simulink model "DiscreteDiscrete"  (R2017b)
settings: Solver=VariableStepAuto  StartTime=0.0  StopTime=10.0  RelTol=1e-3
values from neighbouring files (symbols this model uses):
  kd = double(kd)    [DiscreteDiscreteMatlab.m]    (also in P_I_D.m = eval(S.kd))
  ki = double(ki)    [DiscreteDiscreteEj2Matlab.m]    (also in DiscreteDiscreteMatlab.m; P_I_D.m = eval(S.ki))
  kp = 0    [DiscreteDiscreteEj2Matlab.m]    (also in DiscreteDiscreteMatlab.m = double(kp); P_I_D.m = eval(S.kp))
  r0 = x(3)    [DiscreteDiscreteMatlab.m]
  r1 = x(2)    [DiscreteDiscreteEj2Matlab.m]    (also in DiscreteDiscreteMatlab.m = x(4))
  r2 = x(3)    [DiscreteDiscreteEj2Matlab.m]    (also in DiscreteDiscreteMatlab.m = x(5))
  s0 = x(2)    [DiscreteDiscreteMatlab.m]
  tm = 0.125    [DiscreteDiscreteEj2Matlab.m]    (also in DiscreteDiscreteMatlab.m = 0.25)
libraries: simulink x4
settings Model: Creator=Cx001la  LastModifiedBy=Cx001la

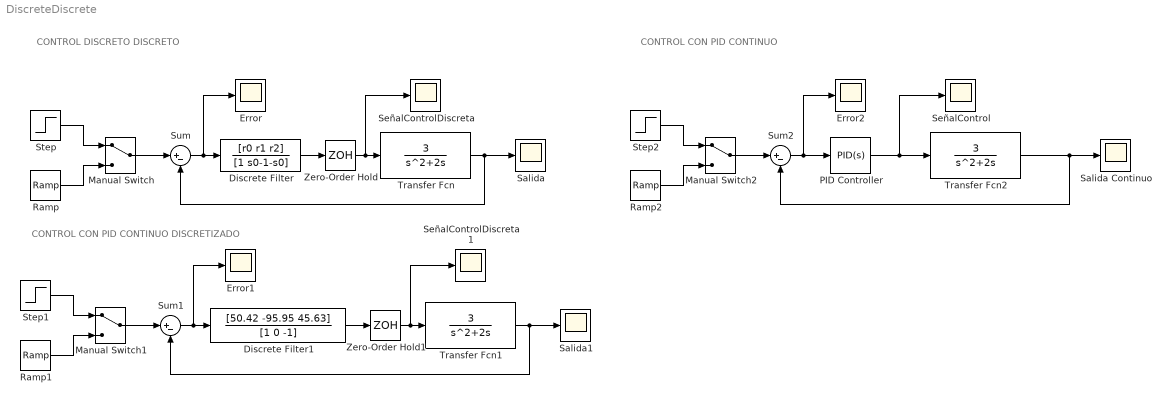
== system DiscreteDiscrete ==
  note: CONTROL CON PID CONTINUO
  note: CONTROL CON PID CONTINUO DISCRETIZADO
  note: CONTROL DISCRETO DISCRETO
  Discrete Filter : DiscreteFilter  Numerator=[r0 r1 r2]  Denominator=[1 s0-1-s0]  SampleTime=tm
  Discrete Filter1 : DiscreteFilter  Numerator=[50.42 -95.95 45.63]  Denominator=[1 0 -1]  SampleTime=0.05%tm
  Error : Scope
  Error1 : Scope
  Error2 : Scope
  Manual Switch : ManualSwitch
  Manual Switch1 : ManualSwitch
  Manual Switch2 : ManualSwitch
  PID Controller : simulink/Continuous/PID Controller  Controller=PID  TimeDomain=Continuous-time  SampleTime=-1  IntegratorMethod=Forward Euler  FilterMethod=Forward Euler  Form=Parallel  UseFilter=on  ControllerParametersSource=internal  P=kp  I=ki  D=kd  N=100  InitialConditionSource=internal  InitialConditionForIntegrator=0  InitialConditionForFilter=0  ExternalReset=none  LimitOutput=off  UpperSaturationLimit=inf  LowerSaturationLimit=-inf  LinearizeAsGain=on  AntiWindupMode=none  Kb=1  TrackingMode=off  Kt=1  PParamMin=[]  PParamMax=[]  IParamMin=[]  IParamMax=[]  DParamMin=[]  DParamMax=[]  NParamMin=[]  NParamMax=[]  KbParamMin=[]  KbParamMax=[]  KtParamMin=[]  KtParamMax=[]  POutMin=[]  POutMax=[]  IOutMin=[]  IOutMax=[]  DOutMin=[]  DOutMax=[]  NOutMin=[]  NOutMax=[]  KbOutMin=[]  KbOutMax=[]  KtOutMin=[]  KtOutMax=[]  IntegratorOutMin=[]  IntegratorOutMax=[]  FilterOutMin=[]  FilterOutMax=[]  SumOutMin=[]  SumOutMax=[]  SumI1OutMin=[]  SumI1OutMax=[]  SumI2OutMin=[]  SumI2OutMax=[]  SumI3OutMin=[]  SumI3OutMax=[]  SumDOutMin=[]  SumDOutMax=[]  SaturationOutMin=[]  SaturationOutMax=[]  IntegratorContinuousStateAttributes=''  IntegratorStateMustResolveToSignalObject=off  IntegratorRTWStateStorageClass=Auto  FilterContinuousStateAttributes=''  FilterStateMustResolveToSignalObject=off  FilterRTWStateStorageClass=Auto  DifferentiatorICPrevScaledInput=0  DifferentiatorOutMin=[]  DifferentiatorOutMax=[]  InitialConditionSetting=State (most efficient)  FilterDiffOutCoefMin=[]  FilterDiffOutCoefMax=[]  SumDenOutMin=[]  SumDenOutMax=[]  SumNumOutMin=[]  SumNumOutMax=[]  ReciprocalOutMin=[]  ReciprocalOutMax=[]  DivideOutMin=[]  DivideOutMax=[]  TunerSelectOption=Transfer Function Based (PID Tuner App)
  Ramp : simulink/Sources/Ramp  slope=1  start=0  X0=0
  Ramp1 : simulink/Sources/Ramp  slope=1  start=0  X0=0
  Ramp2 : simulink/Sources/Ramp  slope=1  start=0  X0=0
  Salida : Scope
  "Salida Continuo " : Scope
  Salida1 : Scope
  SeñalControl : Scope
  SeñalControlDiscreta : Scope
  SeñalControlDiscreta1 : Scope
  Step : Step  SampleTime=0
  Step1 : Step  SampleTime=0
  Step2 : Step  SampleTime=0
  Sum : Sum  Inputs=|+-
  Sum1 : Sum  Inputs=|+-
  Sum2 : Sum  Inputs=|+-
  Transfer Fcn : TransferFcn  Numerator=[3]  Denominator=[1 2 0]
  Transfer Fcn1 : TransferFcn  Numerator=[3]  Denominator=[1 2 0]
  Transfer Fcn2 : TransferFcn  Numerator=[3]  Denominator=[1 2 0]
  Zero-Order Hold : ZeroOrderHold  SampleTime=tm
  Zero-Order Hold1 : ZeroOrderHold  SampleTime=0.05%tm
  wires:
  Transfer Fcn/1 -> Salida/1, Sum/2
  Sum/1 -> Error/1, Discrete Filter/1
  Discrete Filter/1 -> Zero-Order Hold/1
  Zero-Order Hold/1 -> SeñalControlDiscreta/1, Transfer Fcn/1
  Manual Switch/1 -> Sum/1
  Ramp/1 -> Manual Switch/2
  Step/1 -> Manual Switch/1
  Step1/1 -> Manual Switch1/1
  Ramp1/1 -> Manual Switch1/2
  Manual Switch1/1 -> Sum1/1
  Zero-Order Hold1/1 -> Transfer Fcn1/1, SeñalControlDiscreta1/1
  Discrete Filter1/1 -> Zero-Order Hold1/1
  Sum1/1 -> Discrete Filter1/1, Error1/1
  Transfer Fcn1/1 -> Sum1/2, Salida1/1
  Transfer Fcn2/1 -> "Salida Continuo "/1, Sum2/2
  Sum2/1 -> PID Controller/1, Error2/1
  PID Controller/1 -> Transfer Fcn2/1, SeñalControl/1
  Manual Switch2/1 -> Sum2/1
  Ramp2/1 -> Manual Switch2/2
  Step2/1 -> Manual Switch2/1
